simulink model "ARI_26_6_VanDerPolOscilator"  (Simulink 7.8)
settings: Solver=ode45  StartTime=0.0  StopTime=50.0  RelTol=1e-6
libraries: simulink x1
settings Model: Creator=Michael  LastModifiedBy=Michael  ExtModeTrigMode=oneshot  ExtModeArmWhenConnect=off
settings DataIOCC: LimitDataPoints=off
settings OptimizationCC: BlockReduction=off  BooleanDataType=off
settings DebuggingCC: SaveWithParameterizedLinksMsg=none  SignalResolutionControl=TryResolveAllWithWarning  SolverPrmCheckMsg=none  MultiTaskDSMMsg=warning  MultiTaskCondExecSysMsg=none  FcnCallInpInsideContextMsg=Use local settings  StrictBusMsg=None
settings HardwareCC: TargetUnknown=on
settings RTWCC: IncludeERTFirstTime=on
settings GRTTargetCC: ModelReferenceCompliant=off  ParMdlRefBuildCompliant=off  CompOptLevelCompliant=off  ConcurrentExecutionCompliant=off  MatFileLogging=off

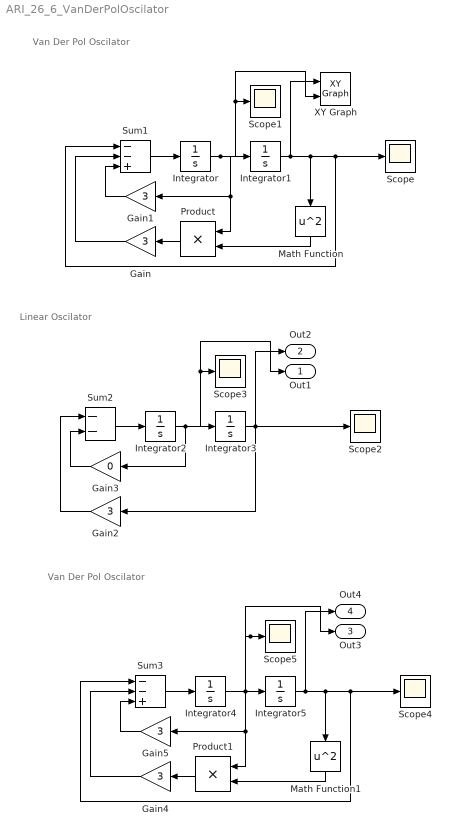
== system ARI_26_6_VanDerPolOscilator ==
  note: Van Der Pol Oscilator
  note: Linear Oscilator
  note: Van Der Pol Oscilator
  Gain{,1..2,4..5} (5 alike) : Gain  Gain=3  SaturateOnIntegerOverflow=on  OutDataTypeStr=Inherit: Same as input  ParamDataTypeStr=Inherit: Same as input
  Gain3 : Gain  Gain=0  SaturateOnIntegerOverflow=on  OutDataTypeStr=Inherit: Same as input  ParamDataTypeStr=Inherit: Same as input
  Integrator : Integrator  InitialCondition=3
  Integrator1 : Integrator  InitialCondition=2
  Integrator2 : Integrator  InitialCondition=1
  Integrator3 : Integrator  InitialCondition=-2:1:2
  Integrator4 : Integrator  InitialCondition=3
  Integrator5 : Integrator  InitialCondition=-2:1:2
  Math Function : Math  Operator=square  SaturateOnIntegerOverflow=on
  Math Function1 : Math  Operator=square  SaturateOnIntegerOverflow=on
  Product : Product  SaturateOnIntegerOverflow=on  RndMeth=Zero  InputSameDT=on  OutDataTypeStr=Inherit: Same as first input
  Product1 : Product  SaturateOnIntegerOverflow=on  RndMeth=Zero  InputSameDT=on  OutDataTypeStr=Inherit: Same as first input
  Scope{,1..5} (6 alike) : Scope
      Scope3 settings: SaveName=ScopeData2
      Scope4 settings: SaveName=ScopeData3
      Scope5 settings: SaveName=ScopeData4
  Sum1 : Sum  Inputs=--+  SaturateOnIntegerOverflow=on  InputSameDT=on  OutDataTypeStr=Inherit: Same as first input
  Sum2 : Sum  Inputs=--  SaturateOnIntegerOverflow=on  InputSameDT=on  OutDataTypeStr=Inherit: Same as first input
  Sum3 : Sum  Inputs=--+  SaturateOnIntegerOverflow=on  InputSameDT=on  OutDataTypeStr=Inherit: Same as first input
  XY Graph : simulink/Sinks/XY Graph  xmin=-3  xmax=3  ymin=-6  ymax=6  st=-1
  Out1 : Outport
  Out2 : Outport  Port=2
  Out3 : Outport  Port=3
  Out4 : Outport  Port=4
  wires:
  Sum1/1 -> Integrator/1
  Integrator/1 -> Integrator1/1, Product/1, Gain1/1, Scope1/1, XY Graph/2
  Math Function/1 -> Product/2
  Product/1 -> Gain/1
  Gain/1 -> Sum1/2
  Gain1/1 -> Sum1/3
  Integrator1/1 -> Math Function/1, Scope/1, Sum1/1, XY Graph/1
  Sum2/1 -> Integrator2/1
  Integrator2/1 -> Scope3/1, Out1/1, Integrator3/1, Gain3/1
  Gain3/1 -> Sum2/2
  Integrator3/1 -> Gain2/1, Scope2/1, Out2/1
  Gain2/1 -> Sum2/1
  Sum3/1 -> Integrator4/1
  Integrator4/1 -> Integrator5/1, Product1/1, Gain5/1, Out3/1, Scope5/1
  Math Function1/1 -> Product1/2
  Product1/1 -> Gain4/1
  Gain4/1 -> Sum3/2
  Gain5/1 -> Sum3/3
  Integrator5/1 -> Math Function1/1, Scope4/1, Sum3/1, Out4/1
